simulink model "chap7_3sim"  (Simulink 7.7)
settings: Solver=ode45  StartTime=0.0  StopTime=10  FixedStep=0.001  RelTol=1e-3
settings Model: Creator=Administrator  LastModifiedBy=ljk  ExtModeTrigMode=oneshot  ExtModeArmWhenConnect=off
settings DataIOCC: LimitDataPoints=off  SignalLoggingName=sigsOut
settings OptimizationCC: BooleanDataType=off  InitFltsAndDblsToZero=on
settings DebuggingCC: SaveWithParameterizedLinksMsg=none  SignalResolutionControl=TryResolveAllWithWarning  SolverPrmCheckMsg=none  MultiTaskDSMMsg=warning  MultiTaskCondExecSysMsg=none  StrictBusMsg=None
settings HardwareCC: TargetUnknown=on
settings RTWCC: IncludeERTFirstTime=on

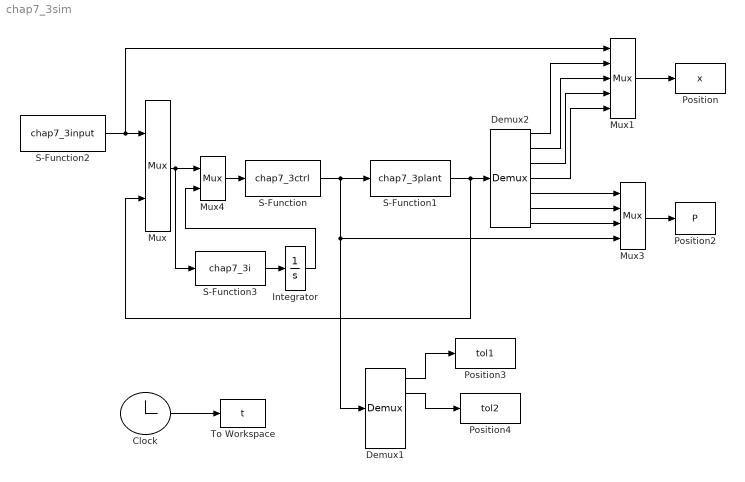
== system chap7_3sim ==
  Clock : Clock
      settings: Decimation=10
  Demux1 : Demux  Outputs=5
  Demux2 : Demux  Outputs=7
  Integrator : Integrator
  Mux : Mux  Inputs=2
  Mux1 : Mux  Inputs=5
  Mux3 : Mux
  Mux4 : Mux  Inputs=2
  Position : ToWorkspace  VariableName=x  SampleTime=-1  SaveFormat=Array
  Position2 : ToWorkspace  VariableName=P  SampleTime=-1  SaveFormat=Array
  Position3 : ToWorkspace  VariableName=tol1  SampleTime=-1  SaveFormat=Array
  Position4 : ToWorkspace  VariableName=tol2  SampleTime=-1  SaveFormat=Array
  S-Function : S-Function  FunctionName=chap7_3ctrl  EnableBusSupport=off
  S-Function1 : S-Function  FunctionName=chap7_3plant  EnableBusSupport=off
  S-Function2 : S-Function  FunctionName=chap7_3input  EnableBusSupport=off
  S-Function3 : S-Function  FunctionName=chap7_3i  EnableBusSupport=off
  To Workspace : ToWorkspace  VariableName=t  SampleTime=-1  SaveFormat=Array
  wires:
  Mux/1 -> S-Function3/1, Mux4/1
  S-Function1/1 -> Demux2/1, Mux/2
  S-Function2/1 -> Mux/1, Mux1/1
  Demux1/1 -> Position3/1
  Demux1/2 -> Position4/1
  S-Function/1 -> S-Function1/1, Mux3/4, Demux1/1
  Mux3/1 -> Position2/1
  Demux2/5 -> Mux3/1
  Mux4/1 -> S-Function/1
  S-Function3/1 -> Integrator/1
  Integrator/1 -> Mux4/2
  Clock/1 -> To Workspace/1
  Mux1/1 -> Position/1
  Demux2/6 -> Mux3/2
  Demux2/7 -> Mux3/3
  Demux2/1 -> Mux1/2
  Demux2/2 -> Mux1/3
  Demux2/3 -> Mux1/4
  Demux2/4 -> Mux1/5
